simulink model "equivalentcircuit"  (R2024b)
settings: Solver=VariableStepAuto  StartTime=0.0  StopTime=tstop  RelTol=1e-3
values from neighbouring files (symbols this model uses):
  bl = 39.4295    [runequivalentcircuit.m]
  re = 6    [runequivalentcircuit.m]
  rf = -1    [runequivalentcircuit.m]
  rms = 15.3849    [runequivalentcircuit.m]
  rr = 2    [runequivalentcircuit.m]
libraries: fl_lib x22, nesl_utility x3
settings Model: Creator=jvermond  LastModifiedBy=jvermond

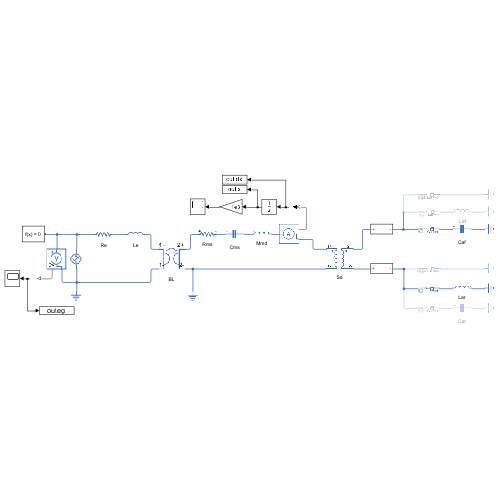
[thumbnail: Simulink's stored preview of the top-level diagram]
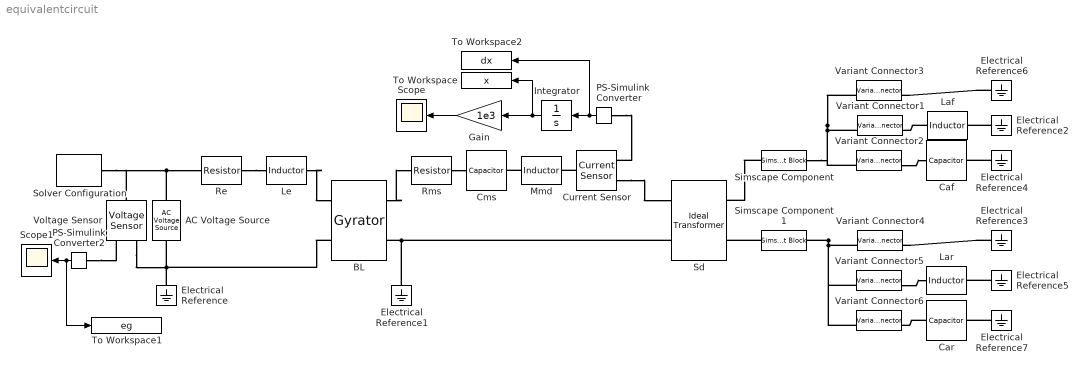
== system equivalentcircuit ==
  AC Voltage Source : fl_lib/Electrical/Electrical Sources/AC Voltage Source  amp=egp V  shift=ps deg  frequency=f Hz
  BL : fl_lib/Electrical/Electrical Elements/Gyrator  G=1/bl 1/Ohm  i1_specify=off  i1_priority=None  i1=0 A  i1_nominal_specify=off  i1_nominal_value=1  i1_nominal_unit=A  v1_specify=off  v1_priority=None  v1=0 V  v1_nominal_specify=off  v1_nominal_value=1  v1_nominal_unit=V  i2_specify=off  i2_priority=None  i2=0 A  i2_nominal_specify=off  i2_nominal_value=1  i2_nominal_unit=A  v2_specify=off  v2_priority=None  v2=0 V  v2_nominal_specify=off  v2_nominal_value=1  v2_nominal_unit=V
      settings: InternalSimscapePortConfiguration="{\"Bottom\":[],\"Left\":[{\"id\":\"p1\",\"label\":\"1+\",\"type\":\"foundation.electrical.electrical\"},{\"id\":\"n1\",\"label\":\"1-\",\"type\":\"foundation.electrical.electrical\"}],\"Right\":[{\"id\":\"p2\",\"label\":\"2+\",\"type\":\"foundation.electrical.electrical\"},{\"id\":\"n2\",\"label\":\"2-\",\"type\":\"foundation.electrical.electrical\"}],\"Top\":[]}"
  Caf : fl_lib/Electrical/Electrical Elements/Capacitor  c=caf F  r=0 Ohm  g=0 1/Ohm  i_specify=off  i_priority=None  i=0 A  i_nominal_specify=off  i_nominal_value=1  i_nominal_unit=A  v_specify=off  v_priority=None  v=0 V  v_nominal_specify=off  v_nominal_value=1  v_nominal_unit=V  vc_specify=off  vc_priority=High  vc=0 V  vc_nominal_specify=off  vc_nominal_value=1  vc_nominal_unit=V
  Car : fl_lib/Electrical/Electrical Elements/Capacitor  c=car F  r=0 Ohm  g=0 1/Ohm  i_specify=off  i_priority=None  i=0 A  i_nominal_specify=off  i_nominal_value=1  i_nominal_unit=A  v_specify=off  v_priority=None  v=0 V  v_nominal_specify=off  v_nominal_value=1  v_nominal_unit=V  vc_specify=off  vc_priority=High  vc=0 V  vc_nominal_specify=off  vc_nominal_value=1  vc_nominal_unit=V
  Cms : fl_lib/Electrical/Electrical Elements/Capacitor  c=cms F  r=0 Ohm  g=0 1/Ohm  i_specify=off  i_priority=None  i=0 A  i_nominal_specify=off  i_nominal_value=1  i_nominal_unit=A  v_specify=off  v_priority=None  v=0 V  v_nominal_specify=off  v_nominal_value=1  v_nominal_unit=V  vc_specify=off  vc_priority=High  vc=0 V  vc_nominal_specify=off  vc_nominal_value=1  vc_nominal_unit=V
  Current Sensor : fl_lib/Electrical/Electrical Sensors/Current Sensor
  Electrical Reference{,1..7} (8 alike) : fl_lib/Electrical/Electrical Elements/Electrical Reference
  Gain : Gain  Gain=1e3
  Integrator : Integrator
  Laf : fl_lib/Electrical/Electrical Elements/Inductor  l=laf H  r=0 Ohm  g=0 1/Ohm  i_specify=off  i_priority=None  i=0 A  i_nominal_specify=off  i_nominal_value=1  i_nominal_unit=A  v_specify=off  v_priority=None  v=0 V  v_nominal_specify=off  v_nominal_value=1  v_nominal_unit=V  i_L_specify=off  i_L_priority=High  i_L=0 A  i_L_nominal_specify=off  i_L_nominal_value=1  i_L_nominal_unit=A
  Lar : fl_lib/Electrical/Electrical Elements/Inductor  l=lar H  r=0 Ohm  g=0 1/Ohm  i_specify=off  i_priority=None  i=0 A  i_nominal_specify=off  i_nominal_value=1  i_nominal_unit=A  v_specify=off  v_priority=None  v=0 V  v_nominal_specify=off  v_nominal_value=1  v_nominal_unit=V  i_L_specify=off  i_L_priority=High  i_L=0 A  i_L_nominal_specify=off  i_L_nominal_value=1  i_L_nominal_unit=A
  Le : fl_lib/Electrical/Electrical Elements/Inductor  l=le H  r=0 Ohm  g=0 1/Ohm  i_specify=off  i_priority=None  i=0 A  i_nominal_specify=off  i_nominal_value=1  i_nominal_unit=A  v_specify=off  v_priority=None  v=0 V  v_nominal_specify=off  v_nominal_value=1  v_nominal_unit=V  i_L_specify=off  i_L_priority=High  i_L=0 A  i_L_nominal_specify=off  i_L_nominal_value=1  i_L_nominal_unit=A
  Mmd : fl_lib/Electrical/Electrical Elements/Inductor  l=mmd H  r=0 Ohm  g=0 1/Ohm  i_specify=off  i_priority=None  i=0 A  i_nominal_specify=off  i_nominal_value=1  i_nominal_unit=A  v_specify=off  v_priority=None  v=0 V  v_nominal_specify=off  v_nominal_value=1  v_nominal_unit=V  i_L_specify=off  i_L_priority=High  i_L=0 A  i_L_nominal_specify=off  i_L_nominal_value=1  i_L_nominal_unit=A
  PS-Simulink Converter : nesl_utility/PS-Simulink Converter  PhysicalDomain=network_engine_domain  SubClassName=ps_output  LeftPortType=input  RightPortType=output  PseudoPeriodic=off  Frequencies=[]  VectorFormat=inherit  Unit=A  AffineConversion=off
  PS-Simulink Converter2 : nesl_utility/PS-Simulink Converter  PhysicalDomain=network_engine_domain  SubClassName=ps_output  LeftPortType=input  RightPortType=output  PseudoPeriodic=off  Frequencies=[]  VectorFormat=inherit  Unit=V  AffineConversion=off
  Re : fl_lib/Electrical/Electrical Elements/Resistor  R=re Ohm  i_specify=off  i_priority=None  i=0 A  i_nominal_specify=off  i_nominal_value=1  i_nominal_unit=A  v_specify=off  v_priority=None  v=0 V  v_nominal_specify=off  v_nominal_value=1  v_nominal_unit=V
  Rms : fl_lib/Electrical/Electrical Elements/Resistor  R=rms Ohm  i_specify=off  i_priority=None  i=0 A  i_nominal_specify=off  i_nominal_value=1  i_nominal_unit=A  v_specify=off  v_priority=None  v=0 V  v_nominal_specify=off  v_nominal_value=1  v_nominal_unit=V
  Scope : Scope
  Scope1 : Scope
  Sd : fl_lib/Electrical/Electrical Elements/Ideal Transformer  n=sd  i1_specify=off  i1_priority=None  i1=0 A  i1_nominal_specify=off  i1_nominal_value=1  i1_nominal_unit=A  v1_specify=off  v1_priority=None  v1=0 V  v1_nominal_specify=off  v1_nominal_value=1  v1_nominal_unit=V  i2_specify=off  i2_priority=None  i2=0 A  i2_nominal_specify=off  i2_nominal_value=1  i2_nominal_unit=A  v2_specify=off  v2_priority=None  v2=0 V  v2_nominal_specify=off  v2_nominal_value=1  v2_nominal_unit=V
  Simscape Component : SimscapeComponentBlock  SourceFile=resistorjv  ComponentPath=resistorjv  ComponentVariants="[\"resistorjv\"]"  ComponentVariantNames="[\"resistorjv\"]"  ClassName=resistorjv  SchemaVersion=1  R=rf Ohm  i_specify=off  i_priority=None  i=0 A  i_nominal_specify=off  i_nominal_value=1  i_nominal_unit=A  v_specify=off  v_priority=None  v=0 V  v_nominal_specify=off  v_nominal_value=1  v_nominal_unit=V
      settings: CopyFcn=simscape.engine.sli.internal.componentblockcallback(gcbh,'COPY')  PreCopyFcn=simscape.engine.sli.internal.componentblockcallback(gcbh,'PRECOPY')  PreDeleteFcn=simscape.engine.sli.internal.componentblockcallback(gcbh,'PREDELETE')  InternalSimscapePortConfiguration="{\"Bottom\":[],\"Left\":[{\"id\":\"p\",\"label\":\"+\",\"type\":\"foundation.electrical.electrical\"}],\"Right\":[{\"id\":\"n\",\"label\":\"-\",\"type\":\"foundation.electrical.electrical\"}],\"Top\":[]}"
      mask Type: Resistor
  Simscape Component1 : SimscapeComponentBlock  SourceFile=resistorjv  ComponentPath=resistorjv  ComponentVariants="[\"resistorjv\"]"  ComponentVariantNames="[\"resistorjv\"]"  ClassName=resistorjv  SchemaVersion=1  R=rr Ohm  i_specify=off  i_priority=None  i=0 A  i_nominal_specify=off  i_nominal_value=1  i_nominal_unit=A  v_specify=off  v_priority=None  v=0 V  v_nominal_specify=off  v_nominal_value=1  v_nominal_unit=V
      settings: CopyFcn=simscape.engine.sli.internal.componentblockcallback(gcbh,'COPY')  PreCopyFcn=simscape.engine.sli.internal.componentblockcallback(gcbh,'PRECOPY')  PreDeleteFcn=simscape.engine.sli.internal.componentblockcallback(gcbh,'PREDELETE')  InternalSimscapePortConfiguration="{\"Bottom\":[],\"Left\":[{\"id\":\"p\",\"label\":\"+\",\"type\":\"foundation.electrical.electrical\"}],\"Right\":[{\"id\":\"n\",\"label\":\"-\",\"type\":\"foundation.electrical.electrical\"}],\"Top\":[]}"
      mask Type: Resistor
  Solver Configuration : nesl_utility/Solver Configuration  PhysicalDomain=network_engine_domain  SubClassName=solver  LeftPortType=input  RightPortType=generic  Tones=[]  Harmonics=[]  SimulateNoise=off  Profile=off  UseLocalSampling=off  EnableSwitchedLinearOptims=on  FrequencyDomain=off  UseCCode=off  RelTol=0.001  AbsTol=0.001  MinStep=1e-09  ToWorkspace=off  RevertToSquareIcSolve=off  NumHomotopyIterations=100  PhasorMode=off  PhasorModeNumHarmonics=1  ConsistencySolver=NEWTON_XTOL_AFTER_FTOL  IndexReductionMethod=DerivativeReplacement  DoDC=off  ResidualTolerance=1e-09  ConsistencyTolSource=GLOBAL  ConsistencyAbsTol=0.001  ConsistencyRelTol=0.001  ConsistencyTolFactor=0.001  UseLocalSolver=off  LocalSolverChoice=NE_BACKWARD_EULER_ADVANCER  ResolveIndetEquations=on  FunctionEvalNumThread=1  LocalSolverSampleTime=0.001  DoFixedCost=off  MaxNonlinIter=3  MaxModeIter=2  ComputeImpulses=off  ImpulseIterations=2  LinearAlgebra=auto  LinearAlgebraNumThread=0  EquationFormulation=NE_TIME_EF  DelaysMemoryBudget=1024  AutomaticFiltering=on  FilteringTimeConstant=0.001  PartitionStorageMethod=AS_NEEDED  PartitionMemoryBudget=1024  PartitionMethod=ROBUST  MultibodyUseLocalSolver=off  MultibodyLocalSolverChoice=ODE1  MultibodyLocalSolverSampleTime=0.001
  To Workspace : ToWorkspace  VariableName=x  SaveFormat=Timeseries  SampleTime=-1
  To Workspace1 : ToWorkspace  VariableName=eg  SaveFormat=Timeseries  SampleTime=-1
  To Workspace2 : ToWorkspace  VariableName=dx  SaveFormat=Timeseries  SampleTime=-1
  Variant Connector1 : VariantPMConnector  VariantControls=__PRM__SERIALIZED__DATA__:Laf==1  ShowConditionOnBlock=on
  Variant Connector2 : VariantPMConnector  VariantControls=__PRM__SERIALIZED__DATA__:Caf==1  ShowConditionOnBlock=on
  Variant Connector3 : VariantPMConnector  VariantControls=__PRM__SERIALIZED__DATA__:Caf==0 && Laf ==0  ShowConditionOnBlock=on
  Variant Connector4 : VariantPMConnector  VariantControls=__PRM__SERIALIZED__DATA__:Car==0 && Lar ==0  ShowConditionOnBlock=on
  Variant Connector5 : VariantPMConnector  VariantControls=__PRM__SERIALIZED__DATA__:Lar==1  ShowConditionOnBlock=on
  Variant Connector6 : VariantPMConnector  VariantControls=__PRM__SERIALIZED__DATA__:Car==1  ShowConditionOnBlock=on
  Voltage Sensor : fl_lib/Electrical/Electrical Sensors/Voltage Sensor
  wires:
  Integrator/1 -> To Workspace/1, Gain/1
  PS-Simulink Converter2/1 -> To Workspace1/1, Scope1/1
  Gain/1 -> Scope/1
  PS-Simulink Converter/1 -> To Workspace2/1, Integrator/1
  connections:
  AC Voltage Source/LConn1 -- Solver Configuration/RConn1 -- Voltage Sensor/LConn1 -- Re/LConn1
  Re/RConn1 -- Le/LConn1
  Le/RConn1 -- BL/LConn1
  BL/LConn2 -- Voltage Sensor/RConn2 -- AC Voltage Source/RConn1 -- Electrical Reference/LConn1
  BL/RConn1 -- Rms/LConn1
  Rms/RConn1 -- Cms/LConn1
  Mmd/LConn1 -- Cms/RConn1
  Sd/LConn2 -- Electrical Reference1/LConn1 -- BL/RConn2
  Simscape Component1/LConn1 -- Sd/RConn2
  Current Sensor/LConn1 -- Mmd/RConn1
  Current Sensor/RConn2 -- Sd/LConn1
  PS-Simulink Converter/LConn1 -- Current Sensor/RConn1
  PS-Simulink Converter2/LConn1 -- Voltage Sensor/RConn1
  Variant Connector1/RConn1 -- Simscape Component/RConn1 -- Variant Connector2/RConn1 -- Variant Connector3/RConn1
  Laf/LConn1 -- Variant Connector1/LConn1
  Variant Connector2/LConn1 -- Caf/LConn1
  Electrical Reference6/LConn1 -- Variant Connector3/LConn1
  Variant Connector4/RConn1 -- Variant Connector6/RConn1 -- Variant Connector5/RConn1 -- Simscape Component1/RConn1
  Variant Connector5/LConn1 -- Lar/LConn1
  Car/LConn1 -- Variant Connector6/LConn1
  Electrical Reference3/LConn1 -- Variant Connector4/LConn1
  Electrical Reference2/LConn1 -- Laf/RConn1
  Electrical Reference4/LConn1 -- Caf/RConn1
  Electrical Reference5/LConn1 -- Lar/RConn1
  Electrical Reference7/LConn1 -- Car/RConn1
  Simscape Component/LConn1 -- Sd/RConn1
